simulink model "gm_sampleModel2045_3_sub"  (R2023a)
settings: Solver=VariableStepAuto  StartTime=0.0  StopTime=10.0  RelTol=1e-3
libraries: hdlsllib x2, simulink x2
settings Model: Creator=user1  LastModifiedBy=user1
settings OptimizationCC: BlockReduction=off  ConditionallyExecuteInputs=off
settings DebuggingCC: InheritedTsInSrcMsg=none

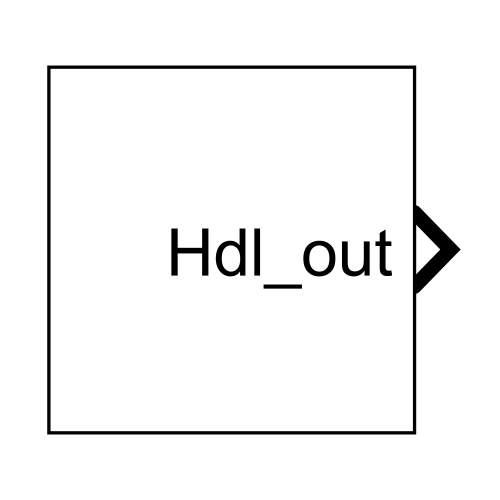
[thumbnail: Simulink's stored preview of the top-level diagram]
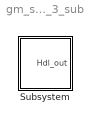
== system gm_sampleModel2045_3_sub ==
  Subsystem : Subsystem

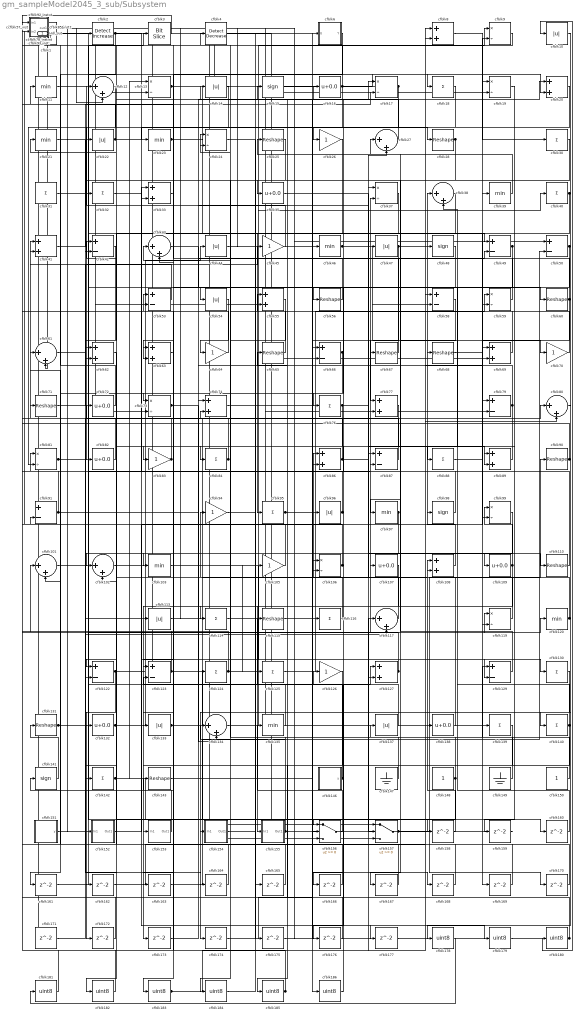
== system gm_sampleModel2045_3_sub/Subsystem ==
  cfblk1 : hdlsllib/Logic and Bit Operations/Bit Shift  mode=Shift Left Logical  N=0
  cfblk{10,14,22,44,47,54,96,113,133,137} (10 alike) : Abs  OutDataTypeStr=uint8  SaturateOnIntegerOverflow=off
  cfblk100_inst : Subsystem
  cfblk{12,27,38,43,61,80,101..102,117,134} (10 alike) : Sum  Inputs=|++  OutDataTypeStr=uint8
  cfblk{11,21,23,39,46,97,103,120,135} (9 alike) : MinMax  OutDataTypeStr=uint8
  cfblk104_inst : Subsystem
  cfblk{26,45,64,70,83,94,105,126} (8 alike) : Gain  OutDataTypeStr=uint8
  cfblk{9,13,17,19,24,37,59,73,81,99,106,119} (12 alike) : Product  Inputs=*/  OutDataTypeStr=uint8  RndMeth=Zero  SaturateOnIntegerOverflow=on
  cfblk{16,35,72,82,107,109,132,138} (8 alike) : Bias  Bias=0.0  SaturateOnIntegerOverflow=off
  cfblk{8,20,33,41,55,62..63,69,74,77,86,89,108,127} (14 alike) : Sum  OutDataTypeStr=uint8
  cfblk{25,28,56,60,65,67..68,71,90,110,115,131,143} (13 alike) : Reshape
  cfblk111_inst : Subsystem
  cfblk112_inst : Subsystem
  cfblk{18,30..32,40,76,84,88,95,114,116,124..125,130,139..140,142} (17 alike) : Sum  Inputs=+  OutDataTypeStr=uint8
  cfblk118_inst : Subsystem
  cfblk{42,49..50,53,58,66,79,87,91,122..123,129} (12 alike) : Sum  Inputs=+-  OutDataTypeStr=uint8
  cfblk128_inst : Subsystem
  cfblk136_inst : Subsystem
  cfblk{15,48,98,141} (4 alike) : Signum
  cfblk146 : Subsystem  mask(Counter Limited){uplimit=double(7), tsamp=double(-1)}
      mask prompts: uplimit "Simulink:masks:UpperLimit_MP"; tsamp "Simulink:masks:SampleTime_MP"
      mask help: Simulink:masks:CounterLimited_MD
      mask init:
      | nbits = double(8);
      | tsamp = double(-1);
      | uplimit = double(7);
  cfblk147 : Ground
  cfblk148 : Constant  OutDataTypeStr=uint8  SampleTime=-1
  cfblk149 : Ground
  cfblk150 : Constant  OutDataTypeStr=uint8  SampleTime=-1
  cfblk151 : Subsystem  mask(Counter Free-Running){NumBits=double(16), tsamp=double(-1)}
      mask prompts: NumBits "Simulink:masks:NumberOfBits_MP"; tsamp "Simulink:masks:SampleTime_MP"
      mask help: Simulink:masks:CounterFreeRunning_MD
  cfblk152 : Subsystem
  cfblk153 : Subsystem
  cfblk154 : Subsystem
  cfblk155 : Subsystem
  cfblk156 : Switch  OutDataTypeStr=uint8  SaturateOnIntegerOverflow=off  InputSameDT=off
  cfblk157 : Switch  OutDataTypeStr=uint8  SaturateOnIntegerOverflow=off  InputSameDT=off
  cfblk{158..177} (20 alike) : Delay  SampleTime=1
  cfblk{178..186} (9 alike) : DataTypeConversion  OutDataTypeStr=uint8  SaturateOnIntegerOverflow=off  RndMeth=Floor
  cfblk2 : simulink/Logic and Bit Operations/Detect Increase  vinit=0.0  OutDataTypeStr=uint8
      settings: LibrarySourceBlock=|
      | hdlsllib/Logic and Bit
      | Operations/Detect
      | Increase
  cfblk3 : hdlsllib/Logic and Bit Operations/Bit Slice  lidx=7  ridx=0
  cfblk34_inst : Subsystem
  cfblk36_inst : Subsystem
  cfblk4 : simulink/Logic and Bit Operations/Detect Decrease  vinit=0.0  OutDataTypeStr=uint8
      settings: LibrarySourceBlock=|
      | hdlsllib/Logic and Bit
      | Operations/Detect
      | Decrease
  cfblk51_inst : Subsystem
  cfblk52_inst : Subsystem
  cfblk57_inst : Subsystem
  cfblk6 : Subsystem  mask(Detect Rise Nonnegative){vinit=double(0), InputProcessing=Elements as channels (sample based), OutDataTypeStr=uint8}
      mask prompts: vinit "Simulink:masks:InitialCondition_MP"; InputProcessing "Simulink:masks:InputProcessing_MP"; OutDataTypeStr "Simulink:masks:OutputDataType_MP"
      mask help: Simulink:masks:DetectRiseNonnegative_MD
      mask init:
      | InputProcessing = 'Elements as channels (sample based)';
      | OutDataTypeStr = 'uint8';
      | vinit = double(0);
      mask TypeOptions InputProcessing: Simulink:masks:ColumnsAsChannelsFrameBased | Simulink:masks:ElementsAsChannelsSampleBased
      mask TypeOptions OutDataTypeStr: Simulink:masks:uint8 | Simulink:masks:boolean
      mask Display: fprintf('U >= 0\n&  NOT\nU/z >= 0')
  cfblk78_inst : Subsystem
  cfblk7_inst : Subsystem
  cfblk85_inst : Subsystem
  cfblk92_inst : Subsystem
  cfblk93_inst : Subsystem
  Hdl_out : Outport  OutDataTypeStr=uint8  SampleTime=1
  wires:
  cfblk1/1 -> cfblk60/1, cfblk20/2, cfblk156/1
  cfblk10/1 -> cfblk178/1
  cfblk100_inst/1(out1) -> cfblk50/1
  cfblk101/1 -> cfblk3/1
  cfblk102/1 -> cfblk44/1
  cfblk103/1 -> cfblk129/2
  cfblk104_inst/1(out1) -> cfblk61/2
  cfblk105/1 -> cfblk4/1
  cfblk106/1 -> cfblk78_inst/2(in2), cfblk7_inst/2(in2)
  cfblk107/1 -> cfblk173/1
  cfblk108/1 -> cfblk38/1
  cfblk109/1 -> cfblk99/1, cfblk155/1(In1)
  cfblk11/1 -> cfblk56/1
  cfblk110/1 -> cfblk16/1
  cfblk111_inst/1(out1) -> cfblk57_inst/1(in1), cfblk73/2
  cfblk112_inst/1(out1) -> cfblk12/2
  cfblk113/1 -> cfblk80/1
  cfblk114/1 -> cfblk9/1
  cfblk115/1 -> cfblk59/1
  cfblk116/1 -> cfblk104_inst/1(in1)
  cfblk117/1 -> cfblk86/1
  cfblk118_inst/1(out1) -> cfblk51_inst/1(in1)
  cfblk119/1 -> cfblk37/2
  cfblk12/1 -> cfblk82/1
  cfblk120/1 -> cfblk94/1, cfblk21/1
  cfblk122/1 -> cfblk172/1, cfblk39/1
  cfblk123/1 -> cfblk72/1, cfblk160/1
  cfblk124/1 -> cfblk85_inst/1(in1), cfblk105/1
  cfblk125/1 -> cfblk98/1
  cfblk126/1 -> cfblk185/1
  cfblk127/1 -> cfblk136_inst/2(in2), cfblk107/1, cfblk101/1
  cfblk128_inst/1(out1) -> cfblk52_inst/2(in2), cfblk48/1, cfblk31/1
  cfblk129/1 -> cfblk25/1
  cfblk13/1 -> cfblk169/1, cfblk95/1
  cfblk130/1 -> cfblk174/1
  cfblk131/1 -> cfblk119/1, cfblk46/1
  cfblk132/1 -> cfblk120/1, cfblk23/1
  cfblk133/1 -> cfblk9/2, cfblk106/2
  cfblk134/1 -> cfblk87/1
  cfblk135/1 -> cfblk53/1
  cfblk136_inst/1(out1) -> cfblk157/3, cfblk13/2, cfblk2/1
  cfblk137/1 -> cfblk106/1
  cfblk138/1 -> cfblk24/1
  cfblk139/1 -> cfblk176/1
  cfblk14/1 -> cfblk73/1
  cfblk140/1 -> cfblk68/1, cfblk153/1(In1)
  cfblk141/1 -> cfblk131/1
  cfblk142/1 -> cfblk165/1, cfblk13/1
  cfblk143/1 -> cfblk66/1
  cfblk146/1(y) -> cfblk74/2, cfblk74/1, cfblk115/1
  cfblk147/1 -> cfblk112_inst/1(in1)
  cfblk148/1 -> cfblk43/1, cfblk182/1
  cfblk149/1 -> cfblk137/1
  cfblk15/1 -> cfblk186/1
  cfblk150/1 -> cfblk129/1
  cfblk151/1(y) -> cfblk127/1
  cfblk152/1(Out1) -> cfblk96/1
  cfblk153/1(Out1) -> cfblk141/1
  cfblk154/1(Out1) -> cfblk108/1
  cfblk155/1(Out1) -> cfblk93_inst/2(in2), cfblk134/1
  cfblk156/1 -> cfblk135/1
  cfblk157/1 -> cfblk90/1, cfblk170/1
  cfblk158/1 -> cfblk108/2
  cfblk159/1 -> cfblk1/1
  cfblk16/1 -> cfblk136_inst/1(in1), cfblk26/1, cfblk18/1
  cfblk160/1 -> cfblk38/2
  cfblk161/1 -> cfblk33/2
  cfblk162/1 -> cfblk8/2
  cfblk163/1 -> cfblk50/2
  cfblk164/1 -> cfblk123/2
  cfblk165/1 -> cfblk42/1
  cfblk166/1 -> cfblk81/1
  cfblk167/1 -> cfblk78_inst/1(in1)
  cfblk168/1 -> cfblk34_inst/2(in2)
  cfblk169/1 -> cfblk91/2
  cfblk17/1 -> cfblk66/2, cfblk63/2, Hdl_out/1
  cfblk170/1 -> cfblk102/2
  cfblk171/1 -> cfblk77/2
  cfblk172/1 -> cfblk85_inst/2(in2)
  cfblk173/1 -> cfblk37/1
  cfblk174/1 -> cfblk86/2
  cfblk175/1 -> cfblk20/1
  cfblk176/1 -> cfblk128_inst/1(in1)
  cfblk177/1 -> cfblk80/2
  cfblk178/1 -> cfblk181/1
  cfblk179/1 -> cfblk10/1
  cfblk18/1 -> cfblk43/2
  cfblk180/1 -> cfblk65/1, cfblk128_inst/2(in2)
  cfblk181/1 -> cfblk92_inst/1(in1)
  cfblk182/1 -> cfblk92_inst/2(in2)
  cfblk183/1 -> cfblk138/1, cfblk117/1
  cfblk184/1 -> cfblk6/1(U)
  cfblk185/1 -> cfblk143/1, cfblk100_inst/1(in1)
  cfblk186/1 -> cfblk126/1
  cfblk19/1 -> cfblk159/1
  cfblk2/1 -> cfblk101/2, cfblk130/1
  cfblk20/1 -> cfblk81/2
  cfblk21/1 -> cfblk122/2
  cfblk22/1 -> cfblk49/1, cfblk28/1, cfblk111_inst/2(in2)
  cfblk23/1 -> cfblk157/2, cfblk156/3
  cfblk24/1 -> cfblk158/1
  cfblk25/1 -> cfblk35/1
  cfblk26/1 -> cfblk62/1
  cfblk27/1 -> cfblk51_inst/2(in2)
  cfblk28/1 -> cfblk42/2, cfblk97/1
  cfblk3/1 -> cfblk7_inst/1(in1)
  cfblk30/1 -> cfblk154/1(In1)
  cfblk31/1 -> cfblk175/1
  cfblk32/1 -> cfblk177/1
  cfblk33/1 -> cfblk123/1
  cfblk34_inst/1(out1) -> cfblk91/1, cfblk69/2
  cfblk35/1 -> cfblk109/1
  cfblk36_inst/1(out1) -> cfblk19/2
  cfblk37/1 -> cfblk133/1
  cfblk38/1 -> cfblk184/1
  cfblk39/1 -> cfblk27/1
  cfblk4/1 -> cfblk179/1
  cfblk40/1 -> cfblk89/2, cfblk54/1
  cfblk41/1 -> cfblk17/2
  cfblk42/1 -> cfblk62/2
  cfblk43/1 -> cfblk59/2
  cfblk44/1 -> cfblk40/1
  cfblk45/1 -> cfblk12/1
  cfblk46/1 -> cfblk58/2, cfblk70/1
  cfblk47/1 -> cfblk77/1, cfblk156/2
  cfblk48/1 -> cfblk76/1
  cfblk49/1 -> cfblk63/1, cfblk103/1
  cfblk50/1 -> cfblk119/2, cfblk88/1
  cfblk51_inst/1(out1) -> cfblk157/1, cfblk171/1
  cfblk52_inst/1(out1) -> cfblk139/1
  cfblk53/1 -> cfblk41/1
  cfblk54/1 -> cfblk64/1
  cfblk55/1 -> cfblk114/1
  cfblk56/1 -> cfblk93_inst/1(in1)
  cfblk57_inst/1(out1) -> cfblk79/2
  cfblk58/1 -> cfblk167/1
  cfblk59/1 -> cfblk11/1
  cfblk6/1(Y) -> cfblk183/1
  cfblk60/1 -> cfblk36_inst/1(in1), cfblk99/2
  cfblk61/1 -> cfblk164/1
  cfblk62/1 -> cfblk122/1
  cfblk63/1 -> cfblk163/1
  cfblk64/1 -> cfblk34_inst/1(in1)
  cfblk65/1 -> cfblk24/2
  cfblk66/1 -> cfblk162/1, cfblk161/1
  cfblk67/1 -> cfblk100_inst/2(in2)
  cfblk68/1 -> cfblk110/1
  cfblk69/1 -> cfblk55/1
  cfblk7_inst/1(out1) -> cfblk152/1(In1)
  cfblk70/1 -> cfblk8/1
  cfblk71/1 -> cfblk45/1
  cfblk72/1 -> cfblk111_inst/1(in1)
  cfblk73/1 -> cfblk69/1, cfblk49/2, cfblk134/2, cfblk17/1
  cfblk74/1 -> cfblk67/1
  cfblk76/1 -> cfblk89/1, cfblk27/2, cfblk84/1
  cfblk77/1 -> cfblk102/1
  cfblk78_inst/1(out1) -> cfblk22/1
  cfblk79/1 -> cfblk58/1, cfblk166/1
  cfblk8/1 -> cfblk30/1
  cfblk80/1 -> cfblk140/1
  cfblk81/1 -> cfblk117/2, cfblk113/1
  cfblk82/1 -> cfblk104_inst/2(in2)
  cfblk83/1 -> cfblk41/2, cfblk32/1
  cfblk84/1 -> cfblk52_inst/1(in1), cfblk118_inst/1(in1)
  cfblk85_inst/1(out1) -> cfblk55/2, cfblk53/2, cfblk125/1
  cfblk86/1 -> cfblk47/1, cfblk14/1
  cfblk87/1 -> cfblk71/1
  cfblk88/1 -> cfblk19/1
  cfblk89/1 -> cfblk83/1
  cfblk9/1 -> cfblk36_inst/2(in2)
  cfblk90/1 -> cfblk33/1, cfblk112_inst/2(in2)
  cfblk91/1 -> cfblk118_inst/2(in2), cfblk124/1
  cfblk92_inst/1(out1) -> cfblk180/1
  cfblk93_inst/1(out1) -> cfblk116/1
  cfblk94/1 -> cfblk87/2
  cfblk95/1 -> cfblk79/1, cfblk168/1
  cfblk96/1 -> cfblk61/1, cfblk57_inst/2(in2)
  cfblk97/1 -> cfblk132/1, cfblk127/2
  cfblk98/1 -> cfblk15/1
  cfblk99/1 -> cfblk142/1

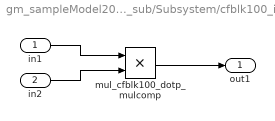
== system gm_sampleModel2045_3_sub/Subsystem/cfblk100_inst ==
  in1 : Inport  OutDataTypeStr=uint8  SampleTime=1
  in2 : Inport  Port=2  OutDataTypeStr=uint8  SampleTime=1
  mul_cfblk100_dotp_mulcomp : Product  Inputs=**  OutDataTypeStr=uint8  SampleTime=1
  out1 : Outport  OutDataTypeStr=uint8  SampleTime=1
  wires:
  in1/1 -> mul_cfblk100_dotp_mulcomp/1
  in2/1 -> mul_cfblk100_dotp_mulcomp/2
  mul_cfblk100_dotp_mulcomp/1 -> out1/1

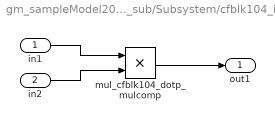
== system gm_sampleModel2045_3_sub/Subsystem/cfblk104_inst ==
  in1 : Inport  OutDataTypeStr=uint8  SampleTime=1
  in2 : Inport  Port=2  OutDataTypeStr=uint8  SampleTime=1
  mul_cfblk104_dotp_mulcomp : Product  Inputs=**  OutDataTypeStr=uint8  SampleTime=1
  out1 : Outport  OutDataTypeStr=uint8  SampleTime=1
  wires:
  in1/1 -> mul_cfblk104_dotp_mulcomp/1
  in2/1 -> mul_cfblk104_dotp_mulcomp/2
  mul_cfblk104_dotp_mulcomp/1 -> out1/1

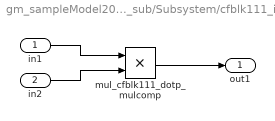
== system gm_sampleModel2045_3_sub/Subsystem/cfblk111_inst ==
  in1 : Inport  OutDataTypeStr=uint8  SampleTime=1
  in2 : Inport  Port=2  OutDataTypeStr=uint8  SampleTime=1
  mul_cfblk111_dotp_mulcomp : Product  Inputs=**  OutDataTypeStr=uint8  SampleTime=1
  out1 : Outport  OutDataTypeStr=uint8  SampleTime=1
  wires:
  in1/1 -> mul_cfblk111_dotp_mulcomp/1
  in2/1 -> mul_cfblk111_dotp_mulcomp/2
  mul_cfblk111_dotp_mulcomp/1 -> out1/1

== system gm_sampleModel2045_3_sub/Subsystem/cfblk112_inst ==
  in1 : Inport  OutDataTypeStr=uint8  SampleTime=1
  in2 : Inport  Port=2  OutDataTypeStr=uint8  SampleTime=1
  mul_cfblk112_dotp_mulcomp : Product  Inputs=**  OutDataTypeStr=uint8  SampleTime=1
  out1 : Outport  OutDataTypeStr=uint8  SampleTime=1
  wires:
  in1/1 -> mul_cfblk112_dotp_mulcomp/1
  in2/1 -> mul_cfblk112_dotp_mulcomp/2
  mul_cfblk112_dotp_mulcomp/1 -> out1/1

== system gm_sampleModel2045_3_sub/Subsystem/cfblk118_inst ==
  in1 : Inport  OutDataTypeStr=uint8  SampleTime=1
  in2 : Inport  Port=2  OutDataTypeStr=uint8  SampleTime=1
  mul_cfblk118_dotp_mulcomp : Product  Inputs=**  OutDataTypeStr=uint8  SampleTime=1
  out1 : Outport  OutDataTypeStr=uint8  SampleTime=1
  wires:
  in1/1 -> mul_cfblk118_dotp_mulcomp/1
  in2/1 -> mul_cfblk118_dotp_mulcomp/2
  mul_cfblk118_dotp_mulcomp/1 -> out1/1

== system gm_sampleModel2045_3_sub/Subsystem/cfblk128_inst ==
  in1 : Inport  OutDataTypeStr=uint8  SampleTime=1
  in2 : Inport  Port=2  OutDataTypeStr=uint8  SampleTime=1
  mul_cfblk128_dotp_mulcomp : Product  Inputs=**  OutDataTypeStr=uint8  SampleTime=1
  out1 : Outport  OutDataTypeStr=uint8  SampleTime=1
  wires:
  in1/1 -> mul_cfblk128_dotp_mulcomp/1
  in2/1 -> mul_cfblk128_dotp_mulcomp/2
  mul_cfblk128_dotp_mulcomp/1 -> out1/1

== system gm_sampleModel2045_3_sub/Subsystem/cfblk136_inst ==
  in1 : Inport  OutDataTypeStr=uint8  SampleTime=1
  in2 : Inport  Port=2  OutDataTypeStr=uint8  SampleTime=1
  mul_cfblk136_dotp_mulcomp : Product  Inputs=**  OutDataTypeStr=uint8  SampleTime=1
  out1 : Outport  OutDataTypeStr=uint8  SampleTime=1
  wires:
  in1/1 -> mul_cfblk136_dotp_mulcomp/1
  in2/1 -> mul_cfblk136_dotp_mulcomp/2
  mul_cfblk136_dotp_mulcomp/1 -> out1/1

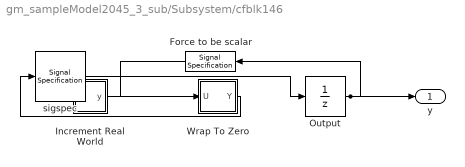
== system gm_sampleModel2045_3_sub/Subsystem/cfblk146 ==
  Force to be scalar : SignalSpecification  DisableCoverage=on  Dimensions=1
  Increment Real World : Subsystem  mask(Real World Value Increment){}
      mask help: Simulink:masks:RealWorldValueIncrement_MD
      mask Display: disp('V++')
  Output : UnitDelay  InitialCondition=0.0  SampleTime=tsamp  HasFrameUpgradeWarning=on
  Wrap To Zero : Subsystem  mask(Wrap To Zero){Threshold=double(7)}
      mask prompts: Threshold "Simulink:masks:Threshold_MP"
      mask help: Simulink:masks:WrapToZero_MD
  sigspec : SignalSpecification  OutDataTypeStr=uint8  Dimensions=1
  y : Outport  SampleTime=1
  wires:
  Force to be scalar/1 -> Increment Real World/1(u)
  Increment Real World/1(y) -> Wrap To Zero/1(U)
  Output/1 -> Force to be scalar/1, y/1
  Wrap To Zero/1(Y) -> sigspec/1
  sigspec/1 -> Output/1

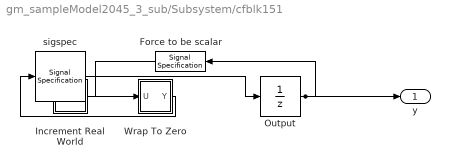
== system gm_sampleModel2045_3_sub/Subsystem/cfblk151 ==
  Force to be scalar : SignalSpecification  DisableCoverage=on  Dimensions=1
  Increment Real World : Subsystem  mask(Real World Value Increment){}
      mask help: Simulink:masks:RealWorldValueIncrement_MD
      mask Display: disp('V++')
  Output : UnitDelay  InitialCondition=0.0  SampleTime=tsamp  HasFrameUpgradeWarning=on
  Wrap To Zero : Subsystem  mask(Wrap To Zero){Threshold=double(65535)}
      mask prompts: Threshold "Simulink:masks:Threshold_MP"
      mask help: Simulink:masks:WrapToZero_MD
  sigspec : SignalSpecification  OutDataTypeStr=uint16  Dimensions=1
  y : Outport  SampleTime=1
  wires:
  Force to be scalar/1 -> Increment Real World/1(u)
  Increment Real World/1(y) -> Wrap To Zero/1(U)
  Output/1 -> Force to be scalar/1, y/1
  Wrap To Zero/1(Y) -> sigspec/1
  sigspec/1 -> Output/1

== system gm_sampleModel2045_3_sub/Subsystem/cfblk152 ==
  In1 : Inport  OutDataTypeStr=uint8  PortDimensions=1  SampleTime=1
  Out1 : Outport  SampleTime=1
  wires:
  In1/1 -> Out1/1

== system gm_sampleModel2045_3_sub/Subsystem/cfblk153 ==
  In1 : Inport  OutDataTypeStr=uint8  PortDimensions=1  SampleTime=1
  Out1 : Outport  SampleTime=1
  wires:
  In1/1 -> Out1/1

== system gm_sampleModel2045_3_sub/Subsystem/cfblk154 ==
  In1 : Inport  OutDataTypeStr=uint8  PortDimensions=1  SampleTime=1
  Out1 : Outport  SampleTime=1
  wires:
  In1/1 -> Out1/1

== system gm_sampleModel2045_3_sub/Subsystem/cfblk155 ==
  In1 : Inport  OutDataTypeStr=uint8  PortDimensions=1  SampleTime=1
  Out1 : Outport  SampleTime=1
  wires:
  In1/1 -> Out1/1

== system gm_sampleModel2045_3_sub/Subsystem/cfblk34_inst ==
  in1 : Inport  OutDataTypeStr=uint8  SampleTime=1
  in2 : Inport  Port=2  OutDataTypeStr=uint8  SampleTime=1
  mul_cfblk34_dotp_mulcomp : Product  Inputs=**  OutDataTypeStr=uint8  SampleTime=1
  out1 : Outport  OutDataTypeStr=uint8  SampleTime=1
  wires:
  in1/1 -> mul_cfblk34_dotp_mulcomp/1
  in2/1 -> mul_cfblk34_dotp_mulcomp/2
  mul_cfblk34_dotp_mulcomp/1 -> out1/1

== system gm_sampleModel2045_3_sub/Subsystem/cfblk36_inst ==
  in1 : Inport  OutDataTypeStr=uint8  SampleTime=1
  in2 : Inport  Port=2  OutDataTypeStr=uint8  SampleTime=1
  mul_cfblk36_dotp_mulcomp : Product  Inputs=**  OutDataTypeStr=uint8  SampleTime=1
  out1 : Outport  OutDataTypeStr=uint8  SampleTime=1
  wires:
  in1/1 -> mul_cfblk36_dotp_mulcomp/1
  in2/1 -> mul_cfblk36_dotp_mulcomp/2
  mul_cfblk36_dotp_mulcomp/1 -> out1/1

== system gm_sampleModel2045_3_sub/Subsystem/cfblk51_inst ==
  in1 : Inport  OutDataTypeStr=uint8  SampleTime=1
  in2 : Inport  Port=2  OutDataTypeStr=uint8  SampleTime=1
  mul_cfblk51_dotp_mulcomp : Product  Inputs=**  OutDataTypeStr=uint8  SampleTime=1
  out1 : Outport  OutDataTypeStr=uint8  SampleTime=1
  wires:
  in1/1 -> mul_cfblk51_dotp_mulcomp/1
  in2/1 -> mul_cfblk51_dotp_mulcomp/2
  mul_cfblk51_dotp_mulcomp/1 -> out1/1

== system gm_sampleModel2045_3_sub/Subsystem/cfblk52_inst ==
  in1 : Inport  OutDataTypeStr=uint8  SampleTime=1
  in2 : Inport  Port=2  OutDataTypeStr=uint8  SampleTime=1
  mul_cfblk52_dotp_mulcomp : Product  Inputs=**  OutDataTypeStr=uint8  SampleTime=1
  out1 : Outport  OutDataTypeStr=uint8  SampleTime=1
  wires:
  in1/1 -> mul_cfblk52_dotp_mulcomp/1
  in2/1 -> mul_cfblk52_dotp_mulcomp/2
  mul_cfblk52_dotp_mulcomp/1 -> out1/1

== system gm_sampleModel2045_3_sub/Subsystem/cfblk57_inst ==
  in1 : Inport  OutDataTypeStr=uint8  SampleTime=1
  in2 : Inport  Port=2  OutDataTypeStr=uint8  SampleTime=1
  mul_cfblk57_dotp_mulcomp : Product  Inputs=**  OutDataTypeStr=uint8  SampleTime=1
  out1 : Outport  OutDataTypeStr=uint8  SampleTime=1
  wires:
  in1/1 -> mul_cfblk57_dotp_mulcomp/1
  in2/1 -> mul_cfblk57_dotp_mulcomp/2
  mul_cfblk57_dotp_mulcomp/1 -> out1/1

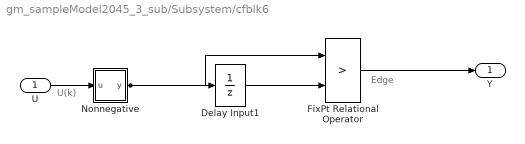
== system gm_sampleModel2045_3_sub/Subsystem/cfblk6 ==
  note: U(k)
  note: Edge
  U : Inport  OutDataTypeStr=uint8  SampleTime=1
  Delay Input1 : UnitDelay  Description=Store in Global RAM  DisableCoverage=on  InitialCondition=vinit  SampleTime=-1  HasFrameUpgradeWarning=on
  FixPt Relational Operator : RelationalOperator  Operator=>  OutDataTypeStr=fixdt(0, 8)  ZeroCross=off  InputSameDT=off
  Nonnegative : Subsystem  mask(Compare To Zero){relop=>=, OutDataTypeStr=boolean, ZeroCross=off}
      mask prompts: relop "Simulink:masks:Operator_MP"; OutDataTypeStr "Simulink:masks:OutputDataType_MP"; ZeroCross "Simulink:masks:EnableZerocrossingDetection_MP"
      mask help: Simulink:masks:CompareToZero_MD
      mask init:
      | OutDataTypeStr = 'boolean';
      | ZeroCross = 'off';
      | blkName = 'sampleModel2045_3_sub/Subsystem/cfblk6/Nonnegative';
      | relop = '>=';
      | setValue = 'boolean';
      mask TypeOptions relop: == | ~= | < | <= | >= | >
      mask TypeOptions OutDataTypeStr: Simulink:masks:uint8 | Simulink:masks:boolean
      mask Callback ZeroCross: sl('zeroCrossEnable', gcbh);
      mask Display: disp([relop,' 0'])
  Y : Outport  SampleTime=1
  wires:
  U/1 -> Nonnegative/1(u)
  Delay Input1/1 -> FixPt Relational Operator/2
  FixPt Relational Operator/1 -> Y/1
  Nonnegative/1(y) -> FixPt Relational Operator/1, Delay Input1/1

== system gm_sampleModel2045_3_sub/Subsystem/cfblk78_inst ==
  in1 : Inport  OutDataTypeStr=uint8  SampleTime=1
  in2 : Inport  Port=2  OutDataTypeStr=uint8  SampleTime=1
  mul_cfblk78_dotp_mulcomp : Product  Inputs=**  OutDataTypeStr=uint8  SampleTime=1
  out1 : Outport  OutDataTypeStr=uint8  SampleTime=1
  wires:
  in1/1 -> mul_cfblk78_dotp_mulcomp/1
  in2/1 -> mul_cfblk78_dotp_mulcomp/2
  mul_cfblk78_dotp_mulcomp/1 -> out1/1

== system gm_sampleModel2045_3_sub/Subsystem/cfblk7_inst ==
  in1 : Inport  OutDataTypeStr=uint8  SampleTime=1
  in2 : Inport  Port=2  OutDataTypeStr=uint8  SampleTime=1
  mul_cfblk7_dotp_mulcomp : Product  Inputs=**  OutDataTypeStr=uint8  SampleTime=1
  out1 : Outport  OutDataTypeStr=uint8  SampleTime=1
  wires:
  in1/1 -> mul_cfblk7_dotp_mulcomp/1
  in2/1 -> mul_cfblk7_dotp_mulcomp/2
  mul_cfblk7_dotp_mulcomp/1 -> out1/1

== system gm_sampleModel2045_3_sub/Subsystem/cfblk85_inst ==
  in1 : Inport  OutDataTypeStr=uint8  SampleTime=1
  in2 : Inport  Port=2  OutDataTypeStr=uint8  SampleTime=1
  mul_cfblk85_dotp_mulcomp : Product  Inputs=**  OutDataTypeStr=uint8  SampleTime=1
  out1 : Outport  OutDataTypeStr=uint8  SampleTime=1
  wires:
  in1/1 -> mul_cfblk85_dotp_mulcomp/1
  in2/1 -> mul_cfblk85_dotp_mulcomp/2
  mul_cfblk85_dotp_mulcomp/1 -> out1/1

== system gm_sampleModel2045_3_sub/Subsystem/cfblk92_inst ==
  in1 : Inport  OutDataTypeStr=uint8  SampleTime=1
  in2 : Inport  Port=2  OutDataTypeStr=uint8  SampleTime=1
  mul_cfblk92_dotp_mulcomp : Product  Inputs=**  OutDataTypeStr=uint8  SampleTime=1
  out1 : Outport  OutDataTypeStr=uint8  SampleTime=1
  wires:
  in1/1 -> mul_cfblk92_dotp_mulcomp/1
  in2/1 -> mul_cfblk92_dotp_mulcomp/2
  mul_cfblk92_dotp_mulcomp/1 -> out1/1

== system gm_sampleModel2045_3_sub/Subsystem/cfblk93_inst ==
  in1 : Inport  OutDataTypeStr=uint8  SampleTime=1
  in2 : Inport  Port=2  OutDataTypeStr=uint8  SampleTime=1
  mul_cfblk93_dotp_mulcomp : Product  Inputs=**  OutDataTypeStr=uint8  SampleTime=1
  out1 : Outport  OutDataTypeStr=uint8  SampleTime=1
  wires:
  in1/1 -> mul_cfblk93_dotp_mulcomp/1
  in2/1 -> mul_cfblk93_dotp_mulcomp/2
  mul_cfblk93_dotp_mulcomp/1 -> out1/1

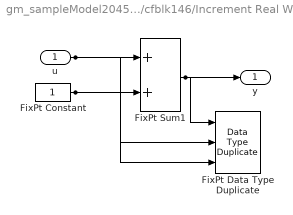
== system gm_sampleModel2045_3_sub/Subsystem/cfblk146/Increment Real World ==
  u : Inport  OutDataTypeStr=uint8  SampleTime=1
  FixPt Constant : Constant  DisableCoverage=on  OutDataTypeStr=Inherit: Inherit via back propagation  SampleTime=-1
  FixPt Data Type Duplicate : DataTypeDuplicate  DisableCoverage=on  NumInputPorts=3
  FixPt Sum1 : Sum  InputSameDT=on  OutDataTypeStr=Inherit: Inherit via back propagation  LockScale=on
  y : Outport  SampleTime=1
  wires:
  u/1 -> FixPt Sum1/1, FixPt Data Type Duplicate/2
  FixPt Constant/1 -> FixPt Sum1/2, FixPt Data Type Duplicate/3
  FixPt Sum1/1 -> FixPt Data Type Duplicate/1, y/1

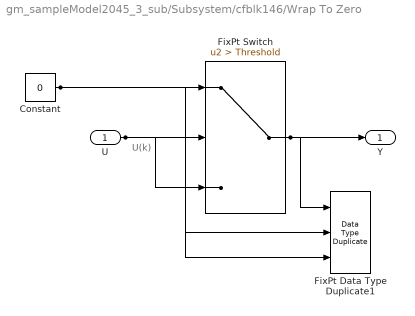
== system gm_sampleModel2045_3_sub/Subsystem/cfblk146/Wrap To Zero ==
  note: U(k)
  U : Inport  OutDataTypeStr=uint8  SampleTime=1
  Constant : Constant  DisableCoverage=on  Value=0  OutDataTypeStr=Inherit: Inherit via back propagation  SampleTime=-1
  FixPt Data Type Duplicate1 : DataTypeDuplicate  DisableCoverage=on  NumInputPorts=3
  FixPt Switch : Switch  Criteria=u2 > Threshold  Threshold=Threshold  OutDataTypeStr=Inherit: Inherit via back propagation  ZeroCross=off  SaturateOnIntegerOverflow=off  InputSameDT=off
  Y : Outport  SampleTime=1
  wires:
  U/1 -> FixPt Switch/3, FixPt Switch/2, FixPt Data Type Duplicate1/2
  Constant/1 -> FixPt Switch/1, FixPt Data Type Duplicate1/3
  FixPt Switch/1 -> FixPt Data Type Duplicate1/1, Y/1

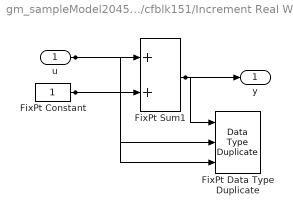
== system gm_sampleModel2045_3_sub/Subsystem/cfblk151/Increment Real World ==
  u : Inport  OutDataTypeStr=uint16  SampleTime=1
  FixPt Constant : Constant  DisableCoverage=on  OutDataTypeStr=Inherit: Inherit via back propagation  SampleTime=-1
  FixPt Data Type Duplicate : DataTypeDuplicate  DisableCoverage=on  NumInputPorts=3
  FixPt Sum1 : Sum  InputSameDT=on  OutDataTypeStr=Inherit: Inherit via back propagation  LockScale=on
  y : Outport  SampleTime=1
  wires:
  u/1 -> FixPt Sum1/1, FixPt Data Type Duplicate/2
  FixPt Constant/1 -> FixPt Sum1/2, FixPt Data Type Duplicate/3
  FixPt Sum1/1 -> FixPt Data Type Duplicate/1, y/1

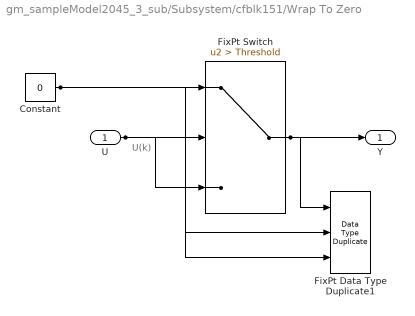
== system gm_sampleModel2045_3_sub/Subsystem/cfblk151/Wrap To Zero ==
  note: U(k)
  U : Inport  OutDataTypeStr=uint16  SampleTime=1
  Constant : Constant  DisableCoverage=on  Value=0  OutDataTypeStr=Inherit: Inherit via back propagation  SampleTime=-1
  FixPt Data Type Duplicate1 : DataTypeDuplicate  DisableCoverage=on  NumInputPorts=3
  FixPt Switch : Switch  Criteria=u2 > Threshold  Threshold=Threshold  OutDataTypeStr=Inherit: Inherit via back propagation  ZeroCross=off  SaturateOnIntegerOverflow=off  InputSameDT=off
  Y : Outport  SampleTime=1
  wires:
  U/1 -> FixPt Switch/3, FixPt Switch/2, FixPt Data Type Duplicate1/2
  Constant/1 -> FixPt Switch/1, FixPt Data Type Duplicate1/3
  FixPt Switch/1 -> FixPt Data Type Duplicate1/1, Y/1

== system gm_sampleModel2045_3_sub/Subsystem/cfblk6/Nonnegative ==
  u : Inport  OutDataTypeStr=uint8  SampleTime=1
  Compare : RelationalOperator  OutDataTypeStr=boolean  ZeroCross=off
  Constant : Constant  DisableCoverage=on  Value=0  OutDataTypeStr=Inherit: Inherit via back propagation  SampleTime=-1  PreserveConstantTs=on
  y : Outport  SampleTime=1
  wires:
  u/1 -> Compare/1
  Compare/1 -> y/1
  Constant/1 -> Compare/2
